simulink model "ECU_Arch"  (R2022b)
settings: Solver=FixedStepDiscrete  StartTime=0.0  StopTime=10.0  RelTol=1e-3
settings Model: Creator=MAAM  LastModifiedBy=MAAM

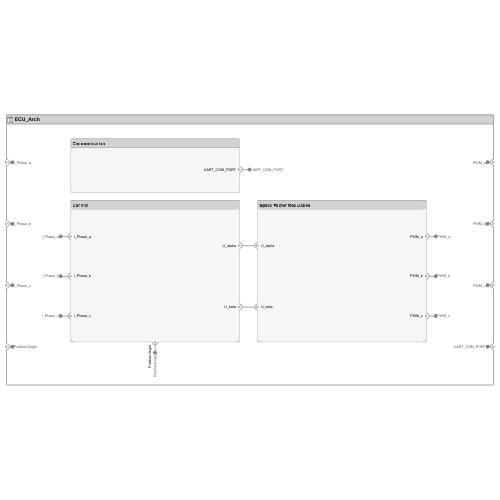
[thumbnail: Simulink's stored preview of the top-level diagram]
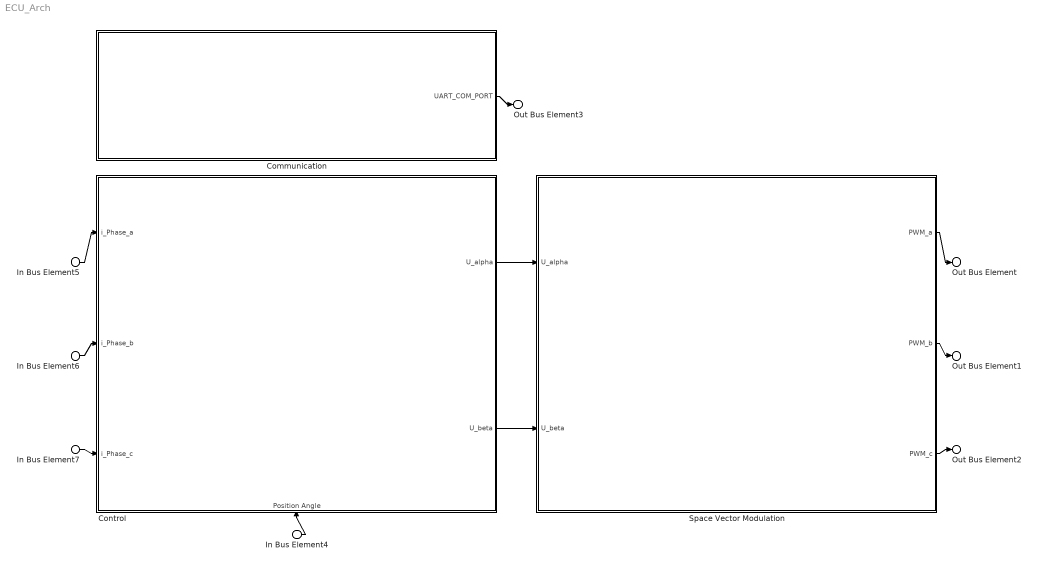
== system ECU_Arch ==
  In Bus Element5 : Inport  PortName=i_Phase_a
  In Bus Element6 : Inport  Port=2  PortName=i_Phase_b
  In Bus Element7 : Inport  Port=3  PortName=i_Phase_c
  In Bus Element4 : Inport  Port=4  PortName=Position Angle
  Communication : Subsystem
      settings: PortSchema="{\"entries\":[{\"content\":{\"headerSize\":26,\"margin\":15,\"minimumSpacing\":25,\"sides\":[{\"content\":{\"connectorIds\":[]},\"type\":\"ConnectorPlacement.EquallySpacedRectSide\",\"uuid\":\"ecb73a61-b18a-4e6f-9a16-a7412467d3dc\"},{\"content\":{\"connectorIds\":[\"Out1\"],\"side\":\"RIGHT\"},\"type\":\"ConnectorPlacement.EquallySpacedRectSide\",\"uuid\":\"05d75da6-23d5-4864-9569-f2b0c11a82bb\"},{\"content\":{\"connectorIds\":[],\"side\":\"TOP\"},\"type\":\"ConnectorPlacement.EquallySpacedRectSide\",\"uuid\":\"f7c561b3-9491-4c59-9ccb-7eaec9c6a3d8\"},{\"content\":{\"connectorIds\":[],\"side\":\"BOTTOM\"},\"type\":\"ConnectorPlacement.EquallySpacedRectSide\",\"uuid\":\"641b09a0-d162-47b4-8d26-f9f12b35e6f7\"}]},\"type\":\"ConnectorPlacement.EquallySpacedConnector\",\"uuid\":\"7fcac072-6609-4f2b-820d-d62cc0efbf31\"}],\"packageUris\":[\"http://schema.mathworks.com/mf0/Connector/R2020b\"],\"version\":\"1.0\"}"
  Control : Subsystem
      settings: PortSchema="{\"entries\":[{\"content\":{\"headerSize\":26,\"margin\":15,\"minimumSpacing\":25,\"sides\":[{\"content\":{\"connectorIds\":[\"In1\",\"In2\",\"In3\"]},\"type\":\"ConnectorPlacement.EquallySpacedRectSide\",\"uuid\":\"ecb73a61-b18a-4e6f-9a16-a7412467d3dc\"},{\"content\":{\"connectorIds\":[\"Out1\",\"Out2\"],\"side\":\"RIGHT\"},\"type\":\"ConnectorPlacement.EquallySpacedRectSide\",\"uuid\":\"05d75da6-23d5-4864-9569-f2b0c11a82bb\"},{\"content\":{\"connectorIds\":[],\"side\":\"TOP\"},\"type\":\"ConnectorPlacement.EquallySpacedRectSide\",\"uuid\":\"f7c561b3-9491-4c59-9ccb-7eaec9c6a3d8\"},{\"content\":{\"connectorIds\":[\"In4\"],\"side\":\"BOTTOM\"},\"type\":\"ConnectorPlacement.EquallySpacedRectSide\",\"uuid\":\"641b09a0-d162-47b4-8d26-f9f12b35e6f7\"}]},\"type\":\"ConnectorPlacement.EquallySpacedConnector\",\"uuid\":\"7fcac072-6609-4f2b-820d-d62cc0efbf31\"}],\"packageUris\":[\"http://schema.mathworks.com/mf0/Connector/R2020b\"],\"version\":\"1.0\"}"
  Space Vector Modulation : Subsystem
      settings: PortSchema="{\"entries\":[{\"content\":{\"headerSize\":26,\"margin\":15,\"minimumSpacing\":25,\"sides\":[{\"content\":{\"connectorIds\":[\"In1\",\"In2\"]},\"type\":\"ConnectorPlacement.EquallySpacedRectSide\",\"uuid\":\"ecb73a61-b18a-4e6f-9a16-a7412467d3dc\"},{\"content\":{\"connectorIds\":[\"Out1\",\"Out2\",\"Out3\"],\"side\":\"RIGHT\"},\"type\":\"ConnectorPlacement.EquallySpacedRectSide\",\"uuid\":\"05d75da6-23d5-4864-9569-f2b0c11a82bb\"},{\"content\":{\"connectorIds\":[],\"side\":\"TOP\"},\"type\":\"ConnectorPlacement.EquallySpacedRectSide\",\"uuid\":\"f7c561b3-9491-4c59-9ccb-7eaec9c6a3d8\"},{\"content\":{\"connectorIds\":[],\"side\":\"BOTTOM\"},\"type\":\"ConnectorPlacement.EquallySpacedRectSide\",\"uuid\":\"baa5380d-922a-4783-9d38-c6d4e2ad9f9d\"}]},\"type\":\"ConnectorPlacement.EquallySpacedConnector\",\"uuid\":\"7fcac072-6609-4f2b-820d-d62cc0efbf31\"}],\"packageUris\":[\"http://schema.mathworks.com/mf0/Connector/R2020b\"],\"version\":\"1.0\"}"
  Out Bus Element : Outport  PortName=PWM_a
  Out Bus Element1 : Outport  Port=2  PortName=PWM_b
  Out Bus Element2 : Outport  Port=3  PortName=PWM_c
  Out Bus Element3 : Outport  Port=4  PortName=UART_COM_PORT
  wires:
  In Bus Element4/1 -> Control/4(Position Angle)
  In Bus Element7/1 -> Control/3(i_Phase_c)
  Communication/1(UART_COM_PORT) -> Out Bus Element3/1
  Space Vector Modulation/1(PWM_a) -> Out Bus Element/1
  Control/2(U_beta) -> Space Vector Modulation/2(U_beta)
  Space Vector Modulation/2(PWM_b) -> Out Bus Element1/1
  In Bus Element6/1 -> Control/2(i_Phase_b)
  In Bus Element5/1 -> Control/1(i_Phase_a)
  Control/1(U_alpha) -> Space Vector Modulation/1(U_alpha)
  Space Vector Modulation/3(PWM_c) -> Out Bus Element2/1

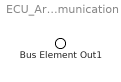
== system ECU_Arch/Communication ==
  Bus Element Out1 : Outport  PortName=UART_COM_PORT

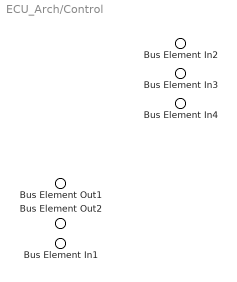
== system ECU_Arch/Control ==
  Bus Element In2 : Inport  PortName=i_Phase_a
  Bus Element In3 : Inport  Port=2  PortName=i_Phase_b
  Bus Element In4 : Inport  Port=3  PortName=i_Phase_c
  Bus Element In1 : Inport  Port=4  PortName=Position Angle
  Bus Element Out1 : Outport  PortName=U_alpha
  Bus Element Out2 : Outport  Port=2  PortName=U_beta

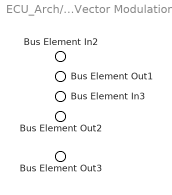
== system ECU_Arch/Space Vector Modulation ==
  Bus Element In2 : Inport  PortName=U_alpha
  Bus Element In3 : Inport  Port=2  PortName=U_beta
  Bus Element Out1 : Outport  PortName=PWM_a
  Bus Element Out2 : Outport  Port=2  PortName=PWM_b
  Bus Element Out3 : Outport  Port=3  PortName=PWM_c
